simulink model "C4_Motorcycle_Analogue_DPDZ"  (R2019b)
settings: Solver=ode45  StartTime=0.0  StopTime=T_sim_motorcycle  MaxStep=dT_sim_sr_max  MinStep=dT_sim_sr_min  RelTol=1e-3
values from neighbouring files (symbols this model uses):
  A_t = r * m * g * sin(theta)    [C2_Preliminary_Controller_Design.m]    (also in D1_Preliminary_Controller_Design.m; D2_Controller_Design.m; D3_PL_Controller_Design.m; D4_DPDZ_Controller_Design.m)
  B_t = r * C_r * m * g    [C2_Preliminary_Controller_Design.m]    (also in D1_Preliminary_Controller_Design.m = 0.0188352; D2_Controller_Design.m = 0.0188352; D3_PL_Controller_Design.m = 0.006309792; D4_DPDZ_Controller_Design.m = 0.006309792)
  c_0 = 1/(m*(h^2))    [C2_Preliminary_Controller_Design.m]    (also in D1_Preliminary_Controller_Design.m = 26.7908045386; D2_Controller_Design.m = 26.7908045386; D3_PL_Controller_Design.m = 79.9725508614; D4_DPDZ_Controller_Design.m = 79.9725508614)
  c_1 = m*g*h    [C2_Preliminary_Controller_Design.m]    (also in D1_Preliminary_Controller_Design.m = 3.790584; D2_Controller_Design.m = 3.790584; D3_PL_Controller_Design.m = 1.26984564; D4_DPDZ_Controller_Design.m = 1.26984564)
  c_2 = m * a * h * sine_lambda/ b    [C2_Preliminary_Controller_Design.m]    (also in D1_Preliminary_Controller_Design.m; D2_Controller_Design.m; D3_PL_Controller_Design.m; D4_DPDZ_Controller_Design.m)
  c_3 = m * a * c * g * sine_lambda/ b    [C2_Preliminary_Controller_Design.m]    (also in D1_Preliminary_Controller_Design.m; D2_Controller_Design.m; D3_PL_Controller_Design.m; D4_DPDZ_Controller_Design.m)
  c_4 = m * h * sine_lambda/ b    [C2_Preliminary_Controller_Design.m]    (also in D1_Preliminary_Controller_Design.m; D2_Controller_Design.m; D3_PL_Controller_Design.m; D4_DPDZ_Controller_Design.m)
  c_5 = h * sine_lambda/ b    [C2_Preliminary_Controller_Design.m]    (also in D1_Preliminary_Controller_Design.m; D2_Controller_Design.m; D3_PL_Controller_Design.m; D4_DPDZ_Controller_Design.m)
  C_t = r * 0.5 * rho_air * C_d * A    [C2_Preliminary_Controller_Design.m]    (also in D1_Preliminary_Controller_Design.m = 3.6e-05; D2_Controller_Design.m = 3.6e-05; D3_PL_Controller_Design.m = 3.6e-05; D4_DPDZ_Controller_Design.m = 3.6e-05)
  c_tv = r/((r.^2) * m + Jaxle)    [C2_Preliminary_Controller_Design.m]    (also in D1_Preliminary_Controller_Design.m; D2_Controller_Design.m; D3_PL_Controller_Design.m; D4_DPDZ_Controller_Design.m)
  d_delta_max = inf * pi/180    (= inf)    [D1_Preliminary_Controller_Design.m]    (also in D2_Controller_Design.m; D3_PL_Controller_Design.m; D4_DPDZ_Controller_Design.m)
  d_phi_0 = 0 * pi/180    (= 0)    [D1_Preliminary_Controller_Design.m]    (also in D2_Controller_Design.m; D3_PL_Controller_Design.m; D4_DPDZ_Controller_Design.m)
  delay_theta = 10    [D1_Preliminary_Controller_Design.m]    (also in D2_Controller_Design.m; D3_PL_Controller_Design.m; D4_DPDZ_Controller_Design.m)
  delta_0 = 0 * pi/180    (= 0)    [D1_Preliminary_Controller_Design.m]    (also in D2_Controller_Design.m; D3_PL_Controller_Design.m; D4_DPDZ_Controller_Design.m)
  delta_max = 70 * pi/180    (= 1.2217304764)    [D1_Preliminary_Controller_Design.m]    (also in D2_Controller_Design.m; D3_PL_Controller_Design.m = 0.610865238198; D4_DPDZ_Controller_Design.m = 0.610865238198)
  eta_g_d = 1    [C2_Preliminary_Controller_Design.m]    (also in D1_Preliminary_Controller_Design.m = 0.95; D2_Controller_Design.m = 0.95; D3_PL_Controller_Design.m = 0.95; D4_DPDZ_Controller_Design.m = 0.95)
  eta_g_s = 1    [C2_Preliminary_Controller_Design.m]    (also in D1_Preliminary_Controller_Design.m = 0.7; D2_Controller_Design.m = 0.8; D3_PL_Controller_Design.m = 0.8; D4_DPDZ_Controller_Design.m = 0.8)
  i_a_max = 1.2    [D1_Preliminary_Controller_Design.m]    (also in D2_Controller_Design.m; D3_PL_Controller_Design.m; D4_DPDZ_Controller_Design.m)
  J_s =     [C2_Preliminary_Controller_Design.m]    (also in D1_Preliminary_Controller_Design.m = 0.0001; D2_Controller_Design.m = 0.0001; D3_PL_Controller_Design.m = 0.0001; D4_DPDZ_Controller_Design.m = 0.0001)
  k_m_d =     [C2_Preliminary_Controller_Design.m]    (also in D1_Preliminary_Controller_Design.m = 0.02; D2_Controller_Design.m = 0.02; D3_PL_Controller_Design.m = 0.02; D4_DPDZ_Controller_Design.m = 0.02)
  k_m_s =     [C2_Preliminary_Controller_Design.m]    (also in D1_Preliminary_Controller_Design.m = 0.0157; D2_Controller_Design.m = 0.0157; D3_PL_Controller_Design.m = 0.0157; D4_DPDZ_Controller_Design.m = 0.0157)
  K_P_d = 25    [D3_PL_Controller_Design.m]    (also in D4_DPDZ_Controller_Design.m)
  K_PL_s = 80    [D1_Preliminary_Controller_Design.m]    (also in D2_Controller_Design.m = 60)
  L_a_d =     [C2_Preliminary_Controller_Design.m]    (also in D1_Preliminary_Controller_Design.m = 0.000278; D2_Controller_Design.m = 0.000278; D3_PL_Controller_Design.m = 0.000278; D4_DPDZ_Controller_Design.m = 0.000278)
  L_a_s =     [C2_Preliminary_Controller_Design.m]    (also in D1_Preliminary_Controller_Design.m = 0.00025; D2_Controller_Design.m = 0.00025; D3_PL_Controller_Design.m = 0.00025; D4_DPDZ_Controller_Design.m = 0.00025)
  n_g_d =     [C2_Preliminary_Controller_Design.m]    (also in D1_Preliminary_Controller_Design.m = 50; D2_Controller_Design.m = 50; D3_PL_Controller_Design.m = 50; D4_DPDZ_Controller_Design.m = 50)
  n_g_s =     [C2_Preliminary_Controller_Design.m]    (also in D1_Preliminary_Controller_Design.m = 12.5; D2_Controller_Design.m = 25; D3_PL_Controller_Design.m = 25; D4_DPDZ_Controller_Design.m = 25)
  phi_0 = 2 * pi/180    (= 0.0349065850399)    [D1_Preliminary_Controller_Design.m]    (also in D2_Controller_Design.m = 0.0872664625997; D3_PL_Controller_Design.m = 0.0872664625997; D4_DPDZ_Controller_Design.m = 0.0872664625997)
  pole_PL_s = -75    [D1_Preliminary_Controller_Design.m]    (also in D2_Controller_Design.m = -50)
  r =     [C2_Preliminary_Controller_Design.m]    (also in D1_Preliminary_Controller_Design.m = 0.06; D2_Controller_Design.m = 0.06; D3_PL_Controller_Design.m = 0.06; D4_DPDZ_Controller_Design.m = 0.06)
  R_a_d =     [C2_Preliminary_Controller_Design.m]    (also in D1_Preliminary_Controller_Design.m = 2.19; D2_Controller_Design.m = 2.19; D3_PL_Controller_Design.m = 2.19; D4_DPDZ_Controller_Design.m = 2.19)
  R_a_s =     [C2_Preliminary_Controller_Design.m]    (also in D1_Preliminary_Controller_Design.m = 3.9; D2_Controller_Design.m = 3.9; D3_PL_Controller_Design.m = 3.9; D4_DPDZ_Controller_Design.m = 3.9)
  V_a_max = 11.1    [D1_Preliminary_Controller_Design.m]    (also in D2_Controller_Design.m; D3_PL_Controller_Design.m; D4_DPDZ_Controller_Design.m)
  v_x_ref = 0.15    [D1_Preliminary_Controller_Design.m]    (also in D2_Controller_Design.m = 0.4; D3_PL_Controller_Design.m = 0.02; D4_DPDZ_Controller_Design.m = 0.02)
  zero_PL_s = -50    [D1_Preliminary_Controller_Design.m]    (also in D2_Controller_Design.m = -35)
undefined symbols (not defined in the file or in its folder): K_DPDZ_r, pole_DPDZ_r1, pole_DPDZ_r2, zero_DPDZ_r1, zero_DPDZ_r2
settings Model: Creator=Conor  LastModifiedBy=Conor Healy
settings DataIOCC: SaveOutput=off  SignalLogging=off  DSMLogging=off  SaveTime=off  ReturnWorkspaceOutputs=off
settings SFSimCC: CustomCodeUndefinedFunction=UseInterfaceOnly

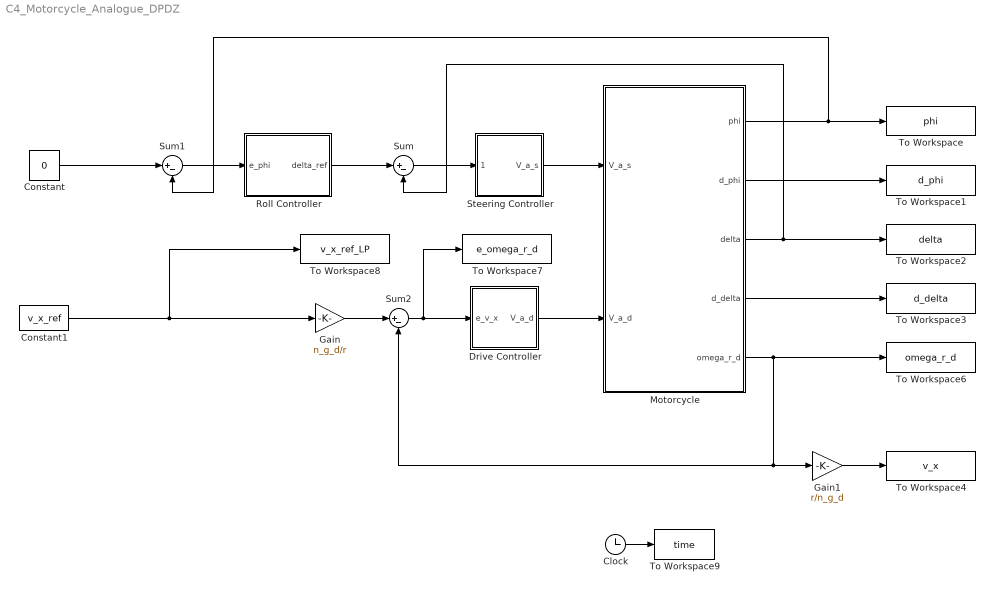
== system C4_Motorcycle_Analogue_DPDZ ==
  Clock : Clock
  Constant : Constant  Value=0
  Constant1 : Constant  Value=v_x_ref
  Drive Controller : Subsystem
  Gain : Gain  Gain=n_g_d/r
      settings: AttributesFormatString=%<Gain>
  Gain1 : Gain  Gain=r/n_g_d
      settings: AttributesFormatString=%<Gain>
  Motorcycle : Subsystem
  Roll Controller : Subsystem
  Steering Controller : Subsystem
  Sum : Sum  Inputs=|+-
  Sum1 : Sum  Inputs=|+-
  Sum2 : Sum  Inputs=|+-
  To Workspace : ToWorkspace  VariableName=phi  SampleTime=-1
  To Workspace1 : ToWorkspace  VariableName=d_phi  SampleTime=-1
  To Workspace2 : ToWorkspace  VariableName=delta  SampleTime=-1
  To Workspace3 : ToWorkspace  VariableName=d_delta  SampleTime=-1
  To Workspace4 : ToWorkspace  VariableName=v_x  SampleTime=-1
  To Workspace6 : ToWorkspace  VariableName=omega_r_d  SampleTime=-1
  To Workspace7 : ToWorkspace  VariableName=e_omega_r_d  SampleTime=-1
  To Workspace8 : ToWorkspace  VariableName=v_x_ref_LP  SampleTime=-1
  To Workspace9 : ToWorkspace  VariableName=time  SampleTime=-1
  wires:
  Motorcycle/1(phi) -> Sum1/2, To Workspace/1
  Motorcycle/3(delta) -> Sum/2, To Workspace2/1
  Constant/1 -> Sum1/1
  Sum1/1 -> Roll Controller/1(e_phi)
  Roll Controller/1(delta_ref) -> Sum/1
  Sum/1 -> Steering Controller/1(e_delta)
  Steering Controller/1(V_a_s) -> Motorcycle/1(V_a_s)
  Motorcycle/2(d_phi) -> To Workspace1/1
  Motorcycle/4(d_delta) -> To Workspace3/1
  Gain1/1 -> To Workspace4/1
  Sum2/1 -> Drive Controller/1(e_v_x), To Workspace7/1
  Motorcycle/5(omega_r_d) -> To Workspace6/1, Gain1/1, Sum2/2
  Gain/1 -> Sum2/1
  Clock/1 -> To Workspace9/1
  Constant1/1 -> To Workspace8/1, Gain/1
  Drive Controller/1(V_a_d) -> Motorcycle/2(V_a_d)

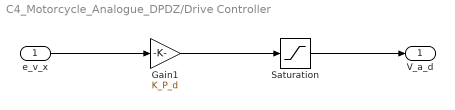
== system C4_Motorcycle_Analogue_DPDZ/Drive Controller ==
  e_v_x : Inport
  Gain1 : Gain  Gain=K_P_d
      settings: AttributesFormatString=%<Gain>
  Saturation : Saturate  UpperLimit=V_a_max  LowerLimit=-V_a_max
  V_a_d : Outport
  wires:
  Saturation/1 -> V_a_d/1
  Gain1/1 -> Saturation/1
  e_v_x/1 -> Gain1/1

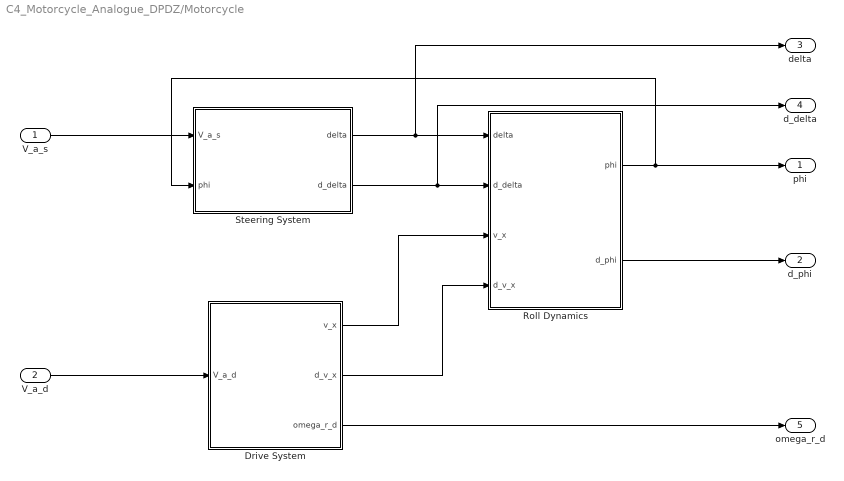
== system C4_Motorcycle_Analogue_DPDZ/Motorcycle ==
  V_a_s : Inport
  V_a_d : Inport  Port=2
  Drive System : Subsystem
  Roll Dynamics : Subsystem
  Steering System : Subsystem
  phi : Outport
  d_phi : Outport  Port=2
  delta : Outport  Port=3
  d_delta : Outport  Port=4
  omega_r_d : Outport  Port=5
  wires:
  Roll Dynamics/1(phi) -> phi/1, Steering System/2(phi)
  Drive System/1(v_x) -> Roll Dynamics/3(v_x)
  Drive System/2(d_v_x) -> Roll Dynamics/4(d_v_x)
  Steering System/2(d_delta) -> d_delta/1, Roll Dynamics/2(d_delta)
  Steering System/1(delta) -> delta/1, Roll Dynamics/1(delta)
  V_a_s/1 -> Steering System/1(V_a_s)
  Roll Dynamics/2(d_phi) -> d_phi/1
  Drive System/3(omega_r_d) -> omega_r_d/1
  V_a_d/1 -> Drive System/1(V_a_d)

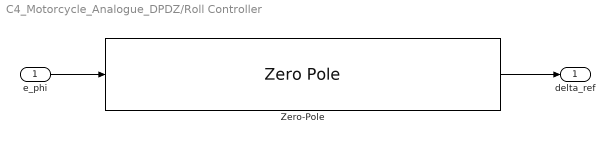
== system C4_Motorcycle_Analogue_DPDZ/Roll Controller ==
  e_phi : Inport
  Zero-Pole : ZeroPole  Zeros=[zero_DPDZ_r1, zero_DPDZ_r2]  Poles=[pole_DPDZ_r1, pole_DPDZ_r2]  Gain=[-K_DPDZ_r]
  delta_ref : Outport
  wires:
  e_phi/1 -> Zero-Pole/1
  Zero-Pole/1 -> delta_ref/1

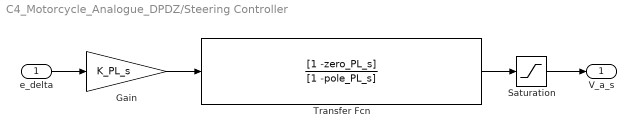
== system C4_Motorcycle_Analogue_DPDZ/Steering Controller ==
  e_delta : Inport
  Gain : Gain  Gain=K_PL_s
  Saturation : Saturate  UpperLimit=V_a_max  LowerLimit=-V_a_max
  Transfer Fcn : TransferFcn  Numerator=[1 -zero_PL_s]  Denominator=[1 -pole_PL_s]
  V_a_s : Outport
  wires:
  Saturation/1 -> V_a_s/1
  e_delta/1 -> Gain/1
  Transfer Fcn/1 -> Saturation/1
  Gain/1 -> Transfer Fcn/1

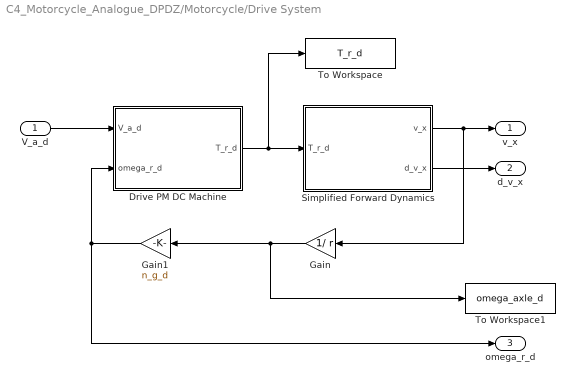
== system C4_Motorcycle_Analogue_DPDZ/Motorcycle/Drive System ==
  V_a_d : Inport
  Drive PM DC Machine : Subsystem
  Gain : Gain  Gain=1/ r
      settings: AttributesFormatString=%<Gain>
  Gain1 : Gain  Gain=n_g_d
      settings: AttributesFormatString=%<Gain>
  Simplified Forward Dynamics : Subsystem
  To Workspace : ToWorkspace  VariableName=T_r_d  SampleTime=-1
  To Workspace1 : ToWorkspace  VariableName=omega_axle_d  SampleTime=-1
  v_x : Outport  VectorParamsAs1DForOutWhenUnconnected=off
  d_v_x : Outport  Port=2  VectorParamsAs1DForOutWhenUnconnected=off
  omega_r_d : Outport  Port=3  VectorParamsAs1DForOutWhenUnconnected=off
  wires:
  Drive PM DC Machine/1(T_r_d) -> To Workspace/1, Simplified Forward Dynamics/1(T_r_d)
  Simplified Forward Dynamics/1(v_x) -> Gain/1, v_x/1
  Simplified Forward Dynamics/2(d_v_x) -> d_v_x/1
  V_a_d/1 -> Drive PM DC Machine/1(V_a_d)
  Gain/1 -> To Workspace1/1, Gain1/1
  Gain1/1 -> omega_r_d/1, Drive PM DC Machine/2(omega_r_d)

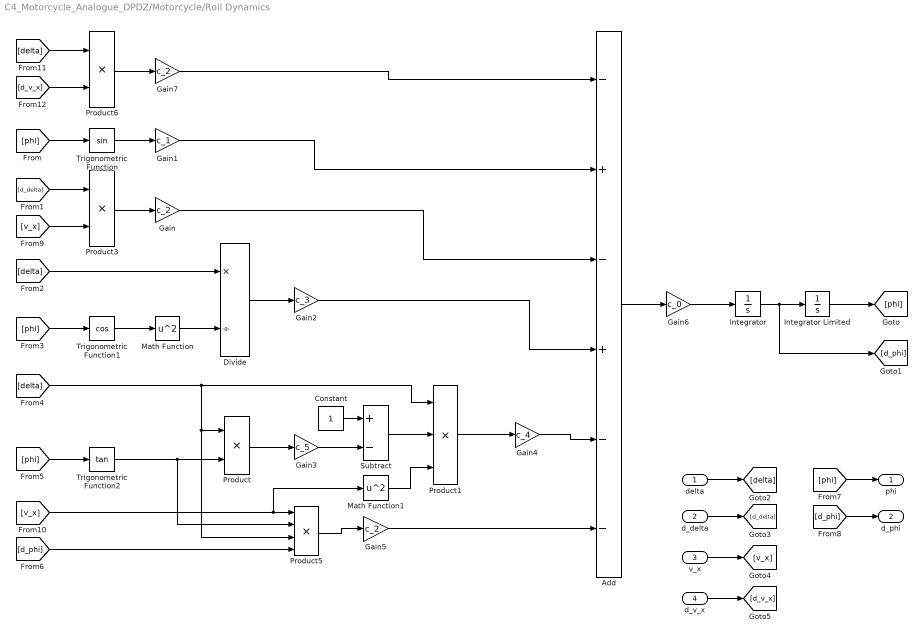
== system C4_Motorcycle_Analogue_DPDZ/Motorcycle/Roll Dynamics ==
  delta : Inport
  d_delta : Inport  Port=2
  v_x : Inport  Port=3
  d_v_x : Inport  Port=4
  Add : Sum  Inputs=-+-+--
  Constant : Constant
  Divide : Product  Inputs=*/
  Gain : Gain  Gain=c_2
  Gain1 : Gain  Gain=c_1
  Gain2 : Gain  Gain=c_3
  Gain3 : Gain  Gain=c_5
  Gain4 : Gain  Gain=c_4
  Gain5 : Gain  Gain=c_2
  Gain6 : Gain  Gain=c_0
  Gain7 : Gain  Gain=c_2
  Integrator : Integrator  InitialCondition=d_phi_0
  Integrator Limited : Integrator  InitialCondition=phi_0  LimitOutput=on  UpperSaturationLimit=pi/2  LowerSaturationLimit=-pi/2
  Math Function : Math  Operator=square  SaturateOnIntegerOverflow=on
  Math Function1 : Math  Operator=square  SaturateOnIntegerOverflow=on
  Product : Product
  Product1 : Product  Inputs=3
  Product3 : Product
  Product5 : Product  Inputs=4
  Product6 : Product
  Subtract : Sum  Inputs=+-
  Trigonometric Function : Trigonometry
  Trigonometric Function1 : Trigonometry  Operator=cos
  Trigonometric Function2 : Trigonometry  Operator=tan
  phi : Outport  VectorParamsAs1DForOutWhenUnconnected=off
  d_phi : Outport  Port=2  VectorParamsAs1DForOutWhenUnconnected=off
  wires:
  Product/1 -> Gain3/1
  Gain2/1 -> Add/4
  Math Function/1 -> Divide/2
  Constant/1 -> Subtract/1
  Trigonometric Function/1 -> Gain1/1
  Gain6/1 -> Integrator/1
  [delta] -> Product5/3, Product/1, Product1/1
  Trigonometric Function2/1 -> Product5/2, Product/2
  [delta] -> Divide/1
  Gain4/1 -> Add/5
  Gain5/1 -> Add/6
  Integrator/1 -> Integrator Limited/1, [d_phi]
  Add/1 -> Gain6/1
  Integrator Limited/1 -> [phi]
  Subtract/1 -> Product1/2
  Gain/1 -> Add/3
  [phi] -> Trigonometric Function/1
  Divide/1 -> Gain2/1
  [phi] -> Trigonometric Function2/1
  [d_phi] -> Product5/4
  Trigonometric Function1/1 -> Math Function/1
  [phi] -> Trigonometric Function1/1
  Gain1/1 -> Add/2
  Gain3/1 -> Subtract/2
  [phi] -> phi/1
  [d_phi] -> d_phi/1
  delta/1 -> [delta]
  d_delta/1 -> [d_delta]
  Product3/1 -> Gain/1
  [d_delta] -> Product3/1
  [v_x] -> Product3/2
  Product1/1 -> Gain4/1
  Math Function1/1 -> Product1/3
  Product5/1 -> Gain5/1
  [v_x] -> Math Function1/1, Product5/1
  v_x/1 -> [v_x]
  d_v_x/1 -> [d_v_x]
  [delta] -> Product6/1
  [d_v_x] -> Product6/2
  Product6/1 -> Gain7/1
  Gain7/1 -> Add/1

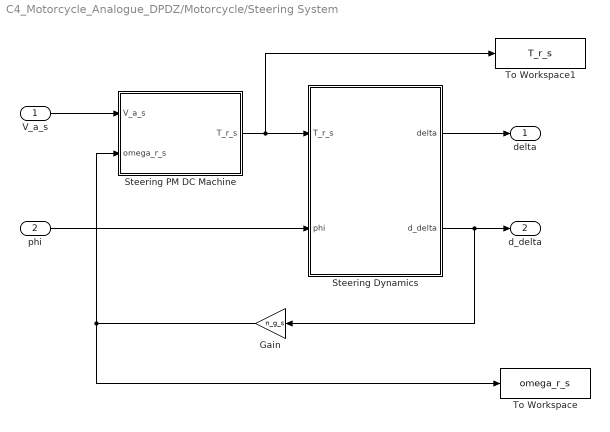
== system C4_Motorcycle_Analogue_DPDZ/Motorcycle/Steering System ==
  V_a_s : Inport
  phi : Inport  Port=2
  Gain : Gain  Gain=n_g_s
      settings: AttributesFormatString=%<Gain>
  Steering Dynamics : Subsystem
  Steering PM DC Machine : Subsystem
  To Workspace : ToWorkspace  VariableName=omega_r_s  SampleTime=-1
  To Workspace1 : ToWorkspace  VariableName=T_r_s  SampleTime=-1
  delta : Outport  VectorParamsAs1DForOutWhenUnconnected=off
  d_delta : Outport  Port=2  VectorParamsAs1DForOutWhenUnconnected=off
  wires:
  Steering Dynamics/2(d_delta) -> d_delta/1, Gain/1
  Gain/1 -> To Workspace/1, Steering PM DC Machine/2(omega_r_s)
  V_a_s/1 -> Steering PM DC Machine/1(V_a_s)
  phi/1 -> Steering Dynamics/2(phi)
  Steering Dynamics/1(delta) -> delta/1
  Steering PM DC Machine/1(T_r_s) -> To Workspace1/1, Steering Dynamics/1(T_r_s)

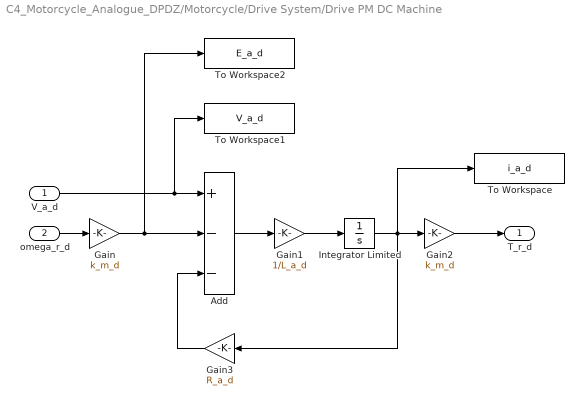
== system C4_Motorcycle_Analogue_DPDZ/Motorcycle/Drive System/Drive PM DC Machine ==
  V_a_d : Inport
  omega_r_d : Inport  Port=2
  Add : Sum  Inputs=+--
  Gain : Gain  Gain=k_m_d
      settings: AttributesFormatString=%<Gain>
  Gain1 : Gain  Gain=1/L_a_d
      settings: AttributesFormatString=%<Gain>
  Gain2 : Gain  Gain=k_m_d
      settings: AttributesFormatString=%<Gain>
  Gain3 : Gain  Gain=R_a_d
      settings: AttributesFormatString=%<Gain>
  Integrator Limited : Integrator  LimitOutput=on  UpperSaturationLimit=i_a_max  LowerSaturationLimit=-i_a_max
  To Workspace : ToWorkspace  VariableName=i_a_d  SampleTime=-1
  To Workspace1 : ToWorkspace  VariableName=V_a_d  SampleTime=-1
  To Workspace2 : ToWorkspace  VariableName=E_a_d  SampleTime=-1
  T_r_d : Outport  VectorParamsAs1DForOutWhenUnconnected=off
  wires:
  V_a_d/1 -> To Workspace1/1, Add/1
  Gain/1 -> To Workspace2/1, Add/2
  omega_r_d/1 -> Gain/1
  Add/1 -> Gain1/1
  Gain1/1 -> Integrator Limited/1
  Integrator Limited/1 -> Gain2/1, To Workspace/1, Gain3/1
  Gain3/1 -> Add/3
  Gain2/1 -> T_r_d/1

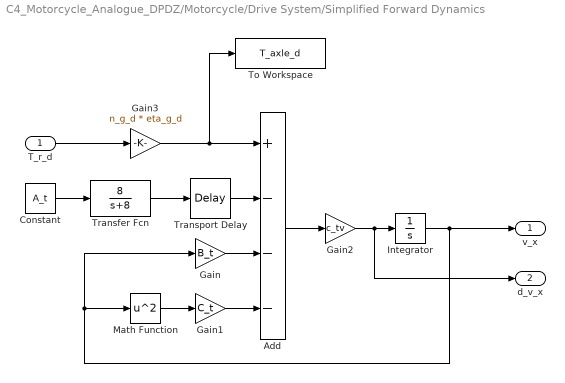
== system C4_Motorcycle_Analogue_DPDZ/Motorcycle/Drive System/Simplified Forward Dynamics ==
  T_r_d : Inport
  Add : Sum  Inputs=+---
  Constant : Constant  Value=A_t
  Gain : Gain  Gain=B_t
  Gain1 : Gain  Gain=C_t
  Gain2 : Gain  Gain=c_tv
  Gain3 : Gain  Gain=n_g_d * eta_g_d
      settings: AttributesFormatString=%<Gain>
  Integrator : Integrator
  Math Function : Math  Operator=square  SaturateOnIntegerOverflow=on
  To Workspace : ToWorkspace  VariableName=T_axle_d  SampleTime=-1
  Transfer Fcn : TransferFcn  Numerator=[8]  Denominator=[1 8]
  Transport Delay : TransportDelay  DelayTime=delay_theta  BufferSize=4096
  v_x : Outport  VectorParamsAs1DForOutWhenUnconnected=off
  d_v_x : Outport  Port=2  VectorParamsAs1DForOutWhenUnconnected=off
  wires:
  Gain/1 -> Add/3
  Gain1/1 -> Add/4
  Gain3/1 -> To Workspace/1, Add/1
  T_r_d/1 -> Gain3/1
  Math Function/1 -> Gain1/1
  Add/1 -> Gain2/1
  Gain2/1 -> d_v_x/1, Integrator/1
  Integrator/1 -> v_x/1, Math Function/1, Gain/1
  Transport Delay/1 -> Add/2
  Constant/1 -> Transfer Fcn/1
  Transfer Fcn/1 -> Transport Delay/1

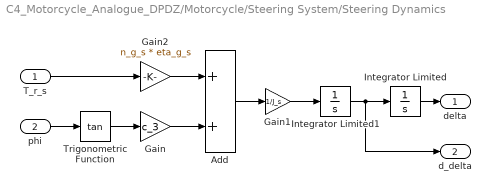
== system C4_Motorcycle_Analogue_DPDZ/Motorcycle/Steering System/Steering Dynamics ==
  T_r_s : Inport
  phi : Inport  Port=2
  Add : Sum
  Gain : Gain  Gain=c_3
  Gain1 : Gain  Gain=1/J_s
      settings: AttributesFormatString=%<Gain>
  Gain2 : Gain  Gain=n_g_s * eta_g_s
      settings: AttributesFormatString=%<Gain>
  Integrator Limited : Integrator  InitialCondition=delta_0  LimitOutput=on  UpperSaturationLimit=delta_max  LowerSaturationLimit=-delta_max
  Integrator Limited1 : Integrator  LimitOutput=on  UpperSaturationLimit=d_delta_max  LowerSaturationLimit=-d_delta_max
  Trigonometric Function : Trigonometry  Operator=tan
  delta : Outport  VectorParamsAs1DForOutWhenUnconnected=off
  d_delta : Outport  Port=2  VectorParamsAs1DForOutWhenUnconnected=off
  wires:
  Gain/1 -> Add/2
  Gain1/1 -> Integrator Limited1/1
  Add/1 -> Gain1/1
  Integrator Limited1/1 -> Integrator Limited/1, d_delta/1
  Trigonometric Function/1 -> Gain/1
  Integrator Limited/1 -> delta/1
  phi/1 -> Trigonometric Function/1
  T_r_s/1 -> Gain2/1
  Gain2/1 -> Add/1

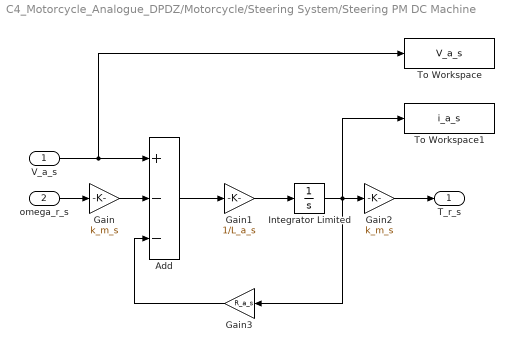
== system C4_Motorcycle_Analogue_DPDZ/Motorcycle/Steering System/Steering PM DC Machine ==
  V_a_s : Inport
  omega_r_s : Inport  Port=2
  Add : Sum  Inputs=+--
  Gain : Gain  Gain=k_m_s
      settings: AttributesFormatString=%<Gain>
  Gain1 : Gain  Gain=1/L_a_s
      settings: AttributesFormatString=%<Gain>
  Gain2 : Gain  Gain=k_m_s
      settings: AttributesFormatString=%<Gain>
  Gain3 : Gain  Gain=R_a_s
      settings: AttributesFormatString=%<Gain>
  Integrator Limited : Integrator  LimitOutput=on  UpperSaturationLimit=i_a_max  LowerSaturationLimit=-i_a_max
  To Workspace : ToWorkspace  VariableName=V_a_s  SampleTime=-1
  To Workspace1 : ToWorkspace  VariableName=i_a_s  SampleTime=-1
  T_r_s : Outport  VectorParamsAs1DForOutWhenUnconnected=off
  wires:
  V_a_s/1 -> To Workspace/1, Add/1
  Gain/1 -> Add/2
  omega_r_s/1 -> Gain/1
  Add/1 -> Gain1/1
  Gain1/1 -> Integrator Limited/1
  Integrator Limited/1 -> To Workspace1/1, Gain3/1, Gain2/1
  Gain3/1 -> Add/3
  Gain2/1 -> T_r_s/1
